simulink model "Cooling_System"  (R2016b)
settings: Solver=FixedStepDiscrete  StartTime=0.0  StopTime=inf  FixedStep=CoolgSys.tiSimnTiStep_C.Value  RelTol=1e-3  EnableMultiTasking=on
settings Model: Creator=djuenema  LastModifiedBy=djuenema
settings DataIOCC: SaveFormat=StructureWithTime  SaveOutput=off  DSMLogging=off  VisualizeSimOutput=off  SaveTime=off  SignalLoggingName=Results
settings OptimizationCC: BlockReduction=off  ConditionallyExecuteInputs=off  LifeSpan=inf
settings DebuggingCC: AllowSymbolicDim=off  SFUnexpectedBacktrackingDiag=warning  SFNoUnconditionalDefaultTransitionDiag=warning  SFExecutionAtInitializationDiag=none
settings ModelReferenceCC: ModelReferenceNumInstancesAllowed=Single  PropagateSignalLabelsOutOfModel=off
settings GRTTargetCC: TargetLangStandard=C89/C90 (ANSI)
settings ConfigComp: CovMetricSettings=dw  CovHtmlReporting=on  CovSaveCumulativeToWorkspaceVar=on  CovSaveSingleToWorkspaceVar=on  CovExternalEMLEnable=off

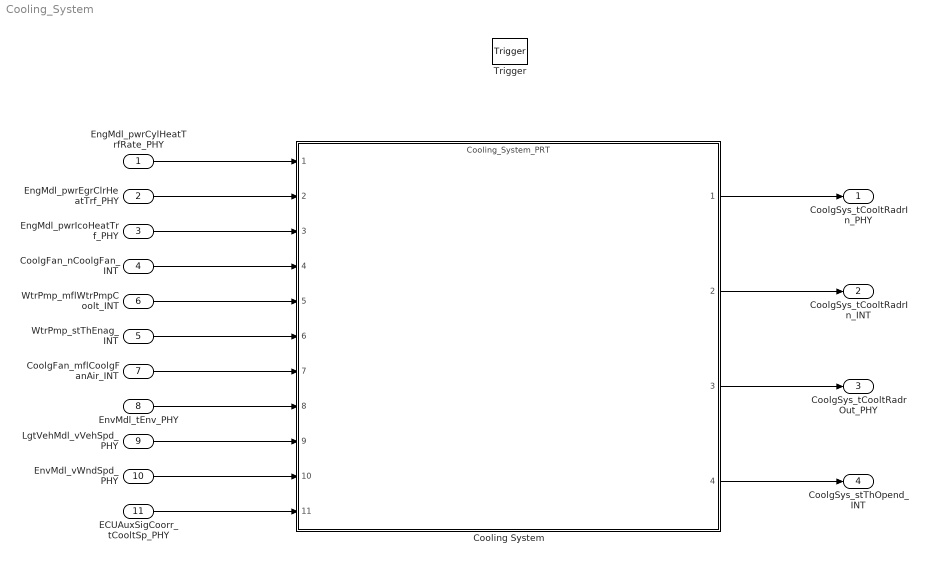
== system Cooling_System ==
  EngMdl_pwrCylHeatTrfRate_PHY : Inport
  EngMdl_pwrEgrClrHeatTrf_PHY : Inport  Port=2
  EngMdl_pwrIcoHeatTrf_PHY : Inport  Port=3
  CoolgFan_nCoolgFan_INT : Inport  Port=4
  WtrPmp_stThEnag_INT : Inport  Port=5
  WtrPmp_mflWtrPmpCoolt_INT : Inport  Port=6
  CoolgFan_mflCoolgFanAir_INT : Inport  Port=7
  EnvMdl_tEnv_PHY : Inport  Port=8
  LgtVehMdl_vVehSpd_PHY : Inport  Port=9
  EnvMdl_vWndSpd_PHY : Inport  Port=10
  ECUAuxSigCoorr_tCooltSp_PHY : Inport  Port=11
  Trigger : TriggerPort  TriggerType=function-call  VariantControl=Variant  PortDimensions=1
  Cooling System : ModelReference  ModelNameDialog=Cooling_System_PRT.slxp  ModelReferenceVersion=1.3  CopyOfModelProtected=on
  CoolgSys_tCooltRadrIn_PHY : Outport
  CoolgSys_tCooltRadrIn_INT : Outport  Port=2
  CoolgSys_tCooltRadrOut_PHY : Outport  Port=3
  CoolgSys_stThOpend_INT : Outport  Port=4
  wires:
  Cooling System/4 -> CoolgSys_stThOpend_INT/1
  Cooling System/3 -> CoolgSys_tCooltRadrOut_PHY/1
  Cooling System/2 -> CoolgSys_tCooltRadrIn_INT/1
  Cooling System/1 -> CoolgSys_tCooltRadrIn_PHY/1
  LgtVehMdl_vVehSpd_PHY/1 -> Cooling System/9
  EnvMdl_tEnv_PHY/1 -> Cooling System/8
  EnvMdl_vWndSpd_PHY/1 -> Cooling System/10
  CoolgFan_nCoolgFan_INT/1 -> Cooling System/4
  EngMdl_pwrCylHeatTrfRate_PHY/1 -> Cooling System/1
  EngMdl_pwrIcoHeatTrf_PHY/1 -> Cooling System/3
  EngMdl_pwrEgrClrHeatTrf_PHY/1 -> Cooling System/2
  CoolgFan_mflCoolgFanAir_INT/1 -> Cooling System/7
  WtrPmp_mflWtrPmpCoolt_INT/1 -> Cooling System/5
  WtrPmp_stThEnag_INT/1 -> Cooling System/6
  ECUAuxSigCoorr_tCooltSp_PHY/1 -> Cooling System/11
